simulink library "fdclib3"  (Simulink 3.00)
undefined symbols (not defined in the file): EM, GM1
libraries: fdclib3 x3, simulink3 x1, fdclib2 x1
settings Model: LastModifiedBy=Dutchroll

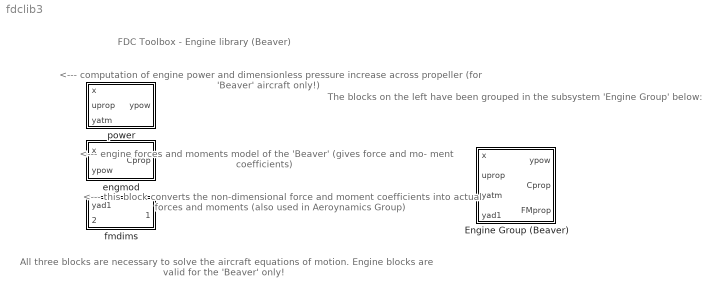
== system fdclib3 ==
  note: FDC Toolbox - Engine library (Beaver)
  note: All three blocks are necessary to solve the aircraft equations
      | of motion. Engine blocks are valid for the 'Beaver' only!
  note: <--- engine forces and moments model
      | of the 'Beaver' (gives force and mo-
      | ment coefficients)
  note: <--- computation of engine power and
      | dimensionless pressure increase across
      | propeller (for 'Beaver' aircraft only!)
  note: <--- this block converts the non-dimensional
      | force and moment coefficients into
      | actual forces and moments
      | (also used in Aeroynamics Group)
  note: The blocks on the left have been grouped
      | in the subsystem 'Engine Group' below:
  Engine Group (Beaver) : Subsystem
  engmod : Subsystem
      mask Type: Engmod
      mask Description: Engine model for the DHC-2 'Beaver'
      mask Help: eval('browse engmod')
      mask Display: disp('Engmod\n(Beaver)')
  fmdims : Subsystem  mask(FMdims){cbar=GM1(1), b=GM1(2), S=GM1(3)}
      mask prompts: cbar "Mean aerodynamic chord [m]:"; b "Wing span [m]:"; S "Wing surface [m^2]:"
      mask help:
      | Calculate forces and moments from
      | dimensionless coefficients.
      mask Help: eval('browse fmdims')
      mask Display: disp('FMdims')
  power : Subsystem
      mask Type: Power
      mask Description:
      | Engine power and dimensionless
      | pressure increase across propeller
      | (model for DHC-2 'Beaver')
      mask Help: eval('browse power')
      mask Display: disp('Power\n(Beaver)')

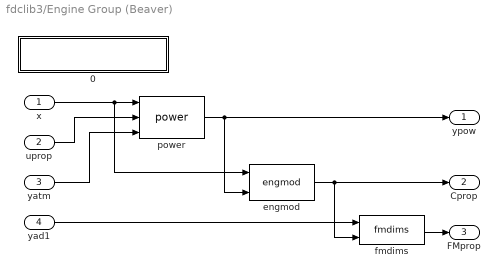
== system fdclib3/Engine Group (Beaver) ==
  x : Inport  Port=1  PortWidth=-1  SampleTime=-1  DataType=auto
      settings: SignalType=auto
  uprop : Inport  Port=2  PortWidth=-1  SampleTime=-1  DataType=auto
      settings: SignalType=auto
  yatm : Inport  Port=3  PortWidth=-1  SampleTime=-1  DataType=auto
      settings: SignalType=auto
  yad1 : Inport  Port=4  PortWidth=-1  SampleTime=-1  DataType=auto
      settings: SignalType=auto
  0 : Subsystem
      settings: OpenFcn=browse enggrp
      mask Display: disp('ENGINE GROUP (level 3)\nM.O. Rauw')
  engmod : fdclib3/engmod
  fmdims : fdclib3/fmdims  cbar=GM1(1)  b=GM1(2)  S=GM1(3)
  power : fdclib3/power
  ypow : Outport  Port=1
  Cprop : Outport  Port=2
  FMprop : Outport  Port=3
  wires:
  yatm/1 -> power/3
  x/1 -> engmod/1, power/1
  yad1/1 -> fmdims/1
  engmod/1 -> fmdims/2, Cprop/1
  fmdims/1 -> FMprop/1
  uprop/1 -> power/2
  power/1 -> engmod/2, ypow/1

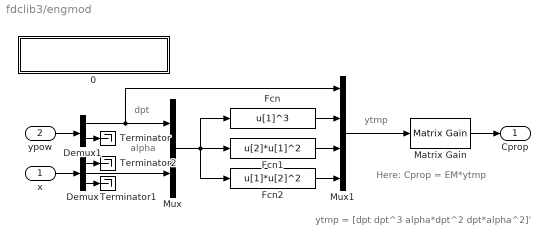
== system fdclib3/engmod ==
  note: ytmp
  note: alpha
  note: dpt
  note: ytmp = [dpt dpt^3 alpha*dpt^2 dpt*alpha^2]'
  note: Here: Cprop = EM*ytmp
  x : Inport  Port=1  PortWidth=-1  SampleTime=-1  DataType=auto
      settings: SignalType=auto
  ypow : Inport  Port=2  PortWidth=-1  SampleTime=-1  DataType=auto
      settings: SignalType=auto
  0 : Subsystem
      settings: OpenFcn=browse engmod
      mask Display: disp('ENGMOD\nM.O. Rauw, March 2003')
  Demux : Demux  Outputs=[1 1 10]
  Demux1 : Demux  Outputs=2
  Fcn : Fcn  Expr=u[1]^3
  Fcn1 : Fcn  Expr=u[2]*u[1]^2
  Fcn2 : Fcn  Expr=u[1]*u[2]^2
  Matrix Gain : simulink3/Math/Matrix Gain  K=EM
  Mux : Mux  Inputs=2
      settings: DisplayOption=none
  Mux1 : Mux  Inputs=4
      settings: DisplayOption=none
  Terminator : Terminator
  Terminator1 : Terminator
  Terminator2 : Terminator
  Cprop : Outport  Port=1
  wires:
  Fcn2/1 -> Mux1/4
  Fcn1/1 -> Mux1/3
  Fcn/1 -> Mux1/2
  Demux1/1 -> Mux1/1, Mux/1
  Mux/1 -> Fcn2/1, Fcn/1, Fcn1/1
  Demux/2 -> Mux/2
  ypow/1 -> Demux1/1
  x/1 -> Demux/1
  Mux1/1 -> Matrix Gain/1
  Matrix Gain/1 -> Cprop/1
  Demux1/2 -> Terminator/1
  Demux/3 -> Terminator1/1
  Demux/1 -> Terminator2/1

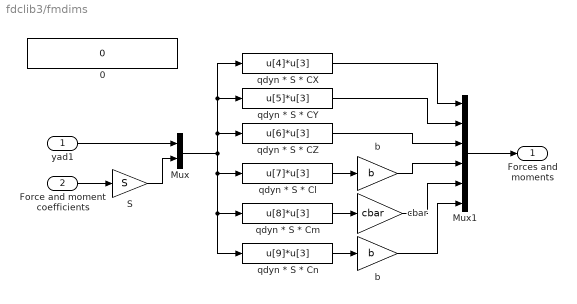
== system fdclib3/fmdims ==
  yad1 : Inport  Port=1  PortWidth=-1  SampleTime=-1  DataType=auto
      settings: SignalType=auto
  Force and moment coefficients : Inport  Port=2  PortWidth=-1  SampleTime=-1  DataType=auto
      settings: SignalType=auto
  0 : fdclib2/fmdims/0
  Mux : Mux  Inputs=[3 6]
      settings: DisplayOption=none
  Mux1 : Mux  Inputs=6
      settings: DisplayOption=none
  S : Gain  Gain=S  SaturateOnIntegerOverflow=on
  b : Gain  Gain=b  SaturateOnIntegerOverflow=on
  "b " : Gain  Gain=b  SaturateOnIntegerOverflow=on
  cbar : Gain  Gain=cbar  SaturateOnIntegerOverflow=on
  qdyn * S * CX : Fcn  Expr=u[4]*u[3]
  qdyn * S * CY : Fcn  Expr=u[5]*u[3]
  qdyn * S * CZ : Fcn  Expr=u[6]*u[3]
  qdyn * S * Cl : Fcn  Expr=u[7]*u[3]
  qdyn * S * Cm : Fcn  Expr=u[8]*u[3]
  qdyn * S * Cn : Fcn  Expr=u[9]*u[3]
  Forces and moments : Outport  Port=1
  wires:
  Mux1/1 -> Forces and moments/1
  "b "/1 -> Mux1/6
  cbar/1 -> Mux1/5
  Force and moment coefficients/1 -> S/1
  Mux/1 -> qdyn * S * CZ/1, qdyn * S * CX/1, qdyn * S * CY/1, qdyn * S * Cl/1, qdyn * S * Cm/1, qdyn * S * Cn/1
  qdyn * S * Cl/1 -> b/1
  qdyn * S * Cm/1 -> cbar/1
  qdyn * S * Cn/1 -> "b "/1
  qdyn * S * CX/1 -> Mux1/1
  qdyn * S * CY/1 -> Mux1/2
  qdyn * S * CZ/1 -> Mux1/3
  b/1 -> Mux1/4
  yad1/1 -> Mux/1
  S/1 -> Mux/2

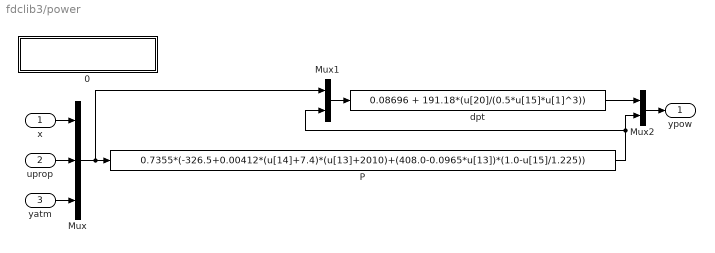
== system fdclib3/power ==
  x : Inport  Port=1  PortWidth=-1  SampleTime=-1  DataType=auto
      settings: SignalType=auto
  uprop : Inport  Port=2  PortWidth=-1  SampleTime=-1  DataType=auto
      settings: SignalType=auto
  yatm : Inport  Port=3  PortWidth=-1  SampleTime=-1  DataType=auto
      settings: SignalType=auto
  0 : Subsystem
      settings: OpenFcn=browse power
      mask Display: disp('POWER\nM.O. Rauw, March 2003')
  Mux : Mux  Inputs=[12 2 5]
      settings: DisplayOption=none
  Mux1 : Mux  Inputs=[19 1]
      settings: DisplayOption=none
  Mux2 : Mux  Inputs=2
      settings: DisplayOption=none
  P : Fcn  Expr=0.7355*(-326.5+0.00412*(u[14]+7.4)*(u[13]+2010)+(408.0-0.0965*u[13])*(1.0-u[15]/1.225))
  dpt : Fcn  Expr=0.08696 + 191.18*(u[20]/(0.5*u[15]*u[1]^3))
  ypow : Outport  Port=1
  wires:
  Mux1/1 -> dpt/1
  P/1 -> Mux1/2, Mux2/2
  Mux/1 -> Mux1/1, P/1
  x/1 -> Mux/1
  uprop/1 -> Mux/2
  yatm/1 -> Mux/3
  dpt/1 -> Mux2/1
  Mux2/1 -> ypow/1

== system fdclib3/Engine Group (Beaver)/0 ==

== system fdclib3/engmod/0 ==

== system fdclib3/power/0 ==
